simulink model "FWBridgeRectifier"  (R2014a)
settings: Solver=ode45  StartTime=0.0  StopTime=0.05  RelTol=1e-3
libraries: fl_lib x8, nesl_utility x2
settings Model: Creator=MuhammadHarris  LastModifiedBy=MuhammadHarris

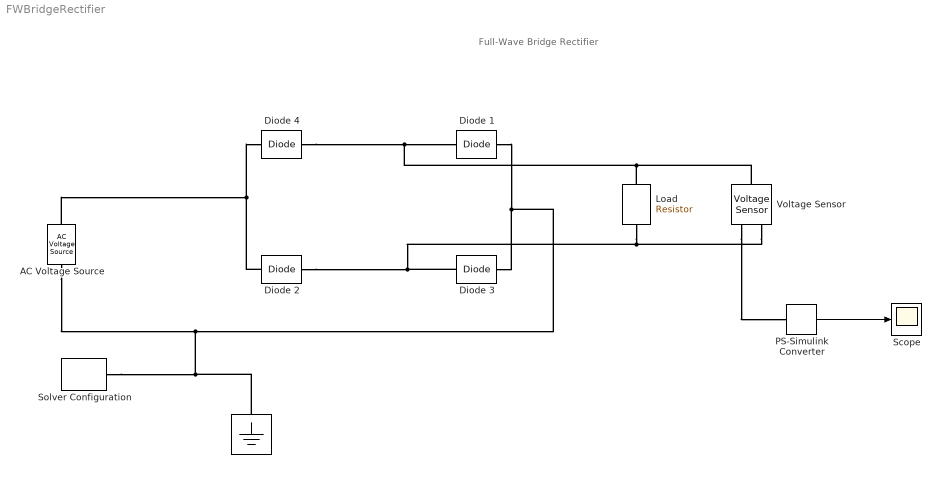
== system FWBridgeRectifier ==
  note: Full-Wave Bridge Rectifier
  " " : fl_lib/Electrical/Electrical Elements/Electrical Reference
  AC Voltage Source : fl_lib/Electrical/Electrical Sources/AC Voltage Source  amp=15 V  shift=0 deg  frequency=60 Hz  omega=0 rad/s
  Diode {1..4} (4 alike) : fl_lib/Electrical/Electrical Elements/Diode  Vf=0.7 V  Ron=0.3 Ohm  Goff=1e-8 1/Ohm  i_specify=off  i_priority=High  i=0 A  v_specify=off  v_priority=High  v=0 V
  Load : fl_lib/Electrical/Electrical Elements/Resistor  R=1 kOhm  i_specify=off  i_priority=High  i=0 A  v_specify=off  v_priority=High  v=0 V
  PS-Simulink Converter : nesl_utility/PS-Simulink Converter  PhysicalDomain=network_engine_domain  SubClassName=ps_output  LeftPortType=input  RightPortType=output  PseudoPeriodic=off  Frequencies=[]  Unit=1  AffineConversion=off
  Scope : Scope
  Solver Configuration : nesl_utility/Solver Configuration  PhysicalDomain=network_engine_domain  SubClassName=solver  LeftPortType=input  RightPortType=generic  Accelerate=off  Tones=[]  Harmonics=[]  SimulateNoise=off  Profile=off  UseLocalSampling=off  EnableSwitchedLinearOptims=on  FrequencyDomain=off  UseCCode=off  RelTol=0.001  AbsTol=1e-06  MinStep=1e-09  ToWorkspace=off  DoDC=off  ResidualTolerance=1e-09  UseLocalSolver=off  LocalSolverChoice=NE_BACKWARD_EULER_ADVANCER  LocalSolverSampleTime=0.001  DoFixedCost=off  MaxNonlinIter=3  MaxModeIter=2  LinearAlgebra=Sparse  DelaysMemoryBudget=1024  AutomaticFiltering=on  FilteringTimeConstant=0.001
  Voltage Sensor : fl_lib/Electrical/Electrical Sensors/Voltage Sensor
  wires:
  PS-Simulink Converter/1 -> Scope/1
  connections:
  Diode 4/RConn1 -- Voltage Sensor/LConn1 -- Load/LConn1 -- Diode 1/RConn1
  Load/RConn1 -- Diode 3/LConn1 -- Diode 2/LConn1 -- Voltage Sensor/RConn2
  Diode 2/RConn1 -- AC Voltage Source/LConn1 -- Diode 4/LConn1
  Diode 1/LConn1 -- Diode 3/RConn1 -- " "/LConn1 -- Solver Configuration/RConn1 -- AC Voltage Source/RConn1
  Voltage Sensor/RConn1 -- PS-Simulink Converter/LConn1
